simulink model "AVI_walking_SLIP"  (R2018a)
settings: Solver=ode45  StartTime=0.0  StopTime=100  MaxStep=1e-3  RelTol=1e-9  AbsTol=1e-6  EnableMultiTasking=on
values from neighbouring files (symbols this model uses):
  a_TD = 64.2076    [AVI_MatLabCode_REIERSEN.m]
  dx_0 = 1.06    [AVI_MatLabCode_REIERSEN.m]
  g = -9.81    [AVI_MatLabCode_REIERSEN.m]
  k = 10000    [AVI_MatLabCode_REIERSEN.m]
  l_0 = 1    [AVI_MatLabCode_REIERSEN.m]
  m = 80    [AVI_MatLabCode_REIERSEN.m]
  No_Steps = 25    [AVI_MatLabCode_REIERSEN.m]
  y_0 = 0.97    [AVI_MatLabCode_REIERSEN.m]
libraries: simulink x6, simulink_extras x1, dspswit3 x1
settings Model: Creator=Work  LastModifiedBy=gyrireiersen
settings SolverCC: AutoScaleAbsTol=off  ZeroCrossAlgorithm=Adaptive
settings DataIOCC: LimitDataPoints=on
settings OptimizationCC: LifeSpan=inf
settings DebuggingCC: AllowSymbolicDim=off  SFUnexpectedBacktrackingDiag=warning  SFNoUnconditionalDefaultTransitionDiag=warning  SFExecutionAtInitializationDiag=none
settings ModelReferenceCC: PropagateSignalLabelsOutOfModel=off
settings CodeAppCC: StateflowObjectComments=on
settings GRTTargetCC: TargetLangStandard=C89/C90 (ANSI)
settings ConfigComp: CovMetricSettings=dw  CovHtmlReporting=on  CovSaveCumulativeToWorkspaceVar=on  CovSaveSingleToWorkspaceVar=on  CovExternalEMLEnable=off

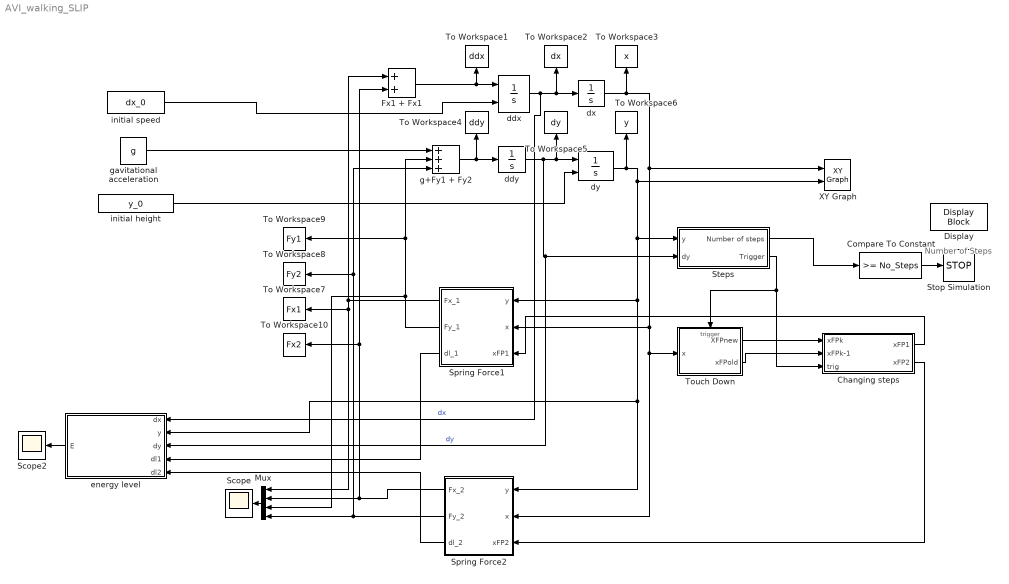
== system AVI_walking_SLIP ==
  note: Number of Steps
  Changing steps : Subsystem
  Compare To Constant : simulink/Logic and Bit Operations/Compare To Constant  relop=>=  const=No_Steps  OutDataTypeStr=boolean
  Display : DisplayBlock  WebBlockId=384  LabelPosition=Hide
  Fx1 + Fx1 : Sum
  Mux : Mux
  Scope : Scope
  Scope2 : Scope
  Spring Force1 : Subsystem
  Spring Force2 : Subsystem
  Steps : Subsystem
  Stop Simulation : Stop
  To Workspace1 : ToWorkspace  VariableName=ddx  SaveFormat=Timeseries  SampleTime=-1
  To Workspace10 : ToWorkspace  VariableName=Fx2  SaveFormat=Timeseries  SampleTime=-1
  To Workspace2 : ToWorkspace  VariableName=dx  SaveFormat=Timeseries  SampleTime=-1
  To Workspace3 : ToWorkspace  VariableName=x  SaveFormat=Timeseries  SampleTime=-1
  To Workspace4 : ToWorkspace  VariableName=ddy  SaveFormat=Timeseries  SampleTime=-1
  To Workspace5 : ToWorkspace  VariableName=dy  SaveFormat=Timeseries  SampleTime=-1
  To Workspace6 : ToWorkspace  VariableName=y  SaveFormat=Timeseries  SampleTime=-1
  To Workspace7 : ToWorkspace  VariableName=Fx1  SaveFormat=Timeseries  SampleTime=-1
  To Workspace8 : ToWorkspace  VariableName=Fy2  SaveFormat=Timeseries  SampleTime=-1
  To Workspace9 : ToWorkspace  VariableName=Fy1  SaveFormat=Timeseries  SampleTime=-1
  Touch Down : Subsystem
  XY Graph : simulink/Sinks/XY Graph  xmin=0  xmax=10  ymin=0  ymax=1.5  st=-1
  ddx : Integrator  InitialConditionSource=external
  ddy : Integrator
  dx : Integrator  LowerSaturationLimit=0
  dy : Integrator  InitialConditionSource=external  LimitOutput=on  LowerSaturationLimit=0
  energy level : Subsystem  TreatAsAtomicUnit=on
  g+Fy1 + Fy2 : Sum  Inputs=+++
  gavitational acceleration : Constant  Value=g
  initial height : Constant  Value=y_0
  initial speed : Constant  Value=dx_0
  wires:
  ddy/1 -> To Workspace5/1, dy/1, energy level/3(dy), Steps/2(dy)  "dy"
  ddx/1 -> To Workspace2/1, dx/1, energy level/1(dx)  "dx"
  gavitational acceleration/1 -> g+Fy1 + Fy2/1
  g+Fy1 + Fy2/1 -> To Workspace4/1, ddy/1
  initial speed/1 -> ddx/2
  initial height/1 -> dy/2
  dy/1 -> To Workspace6/1, Steps/1(y), Spring Force2/1(y), energy level/2(y), Spring Force1/1(y), XY Graph/2
  dx/1 -> Touch Down/1(x), Spring Force2/2(x), Spring Force1/2(x), XY Graph/1, To Workspace3/1
  Compare To Constant/1 -> Stop Simulation/1
  Changing steps/2(xFP2) -> Spring Force2/3(xFP2)
  Steps/1(Number of steps) -> Compare To Constant/1
  Steps/2("Trigger ") -> Touch Down/Trigger, Changing steps/3(trig)
  Touch Down/1(XFPnew) -> Changing steps/1(xFPk)
  Spring Force2/1(Fx_2) -> To Workspace10/1, Fx1 + Fx1/2, Mux/2
  Spring Force1/1(Fx_1) -> Fx1 + Fx1/1, To Workspace7/1, Mux/1
  Mux/1 -> Scope/1
  Changing steps/1(xFP1) -> Spring Force1/3(xFP1)
  Spring Force2/3(dl_2) -> energy level/5(dl2)
  energy level/1(E) -> Scope2/1
  Touch Down/2(xFPold) -> Changing steps/2(xFPk-1)
  Fx1 + Fx1/1 -> To Workspace1/1, ddx/1
  Spring Force1/3("dl_1 ") -> energy level/4(dl1)
  Spring Force2/2(Fy_2) -> To Workspace8/1, g+Fy1 + Fy2/3, Mux/4
  Spring Force1/2(Fy_1) -> Mux/3, g+Fy1 + Fy2/2, To Workspace9/1

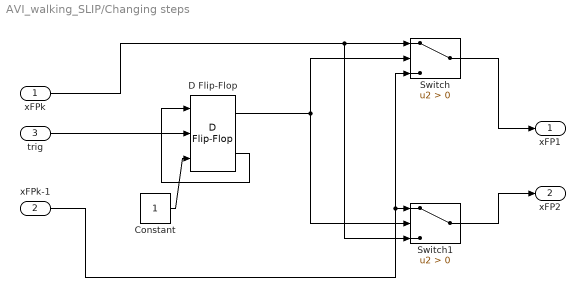
== system AVI_walking_SLIP/Changing steps ==
  xFPk : Inport
  xFPk-1 : Inport  Port=2
  trig : Inport  Port=3
  Constant : Constant
  D Flip-Flop : simulink_extras/Flip Flops/D Flip-Flop
      settings: SourceProductName=Simulink
  Switch : Switch  Criteria=u2 > Threshold
  Switch1 : Switch  Criteria=u2 > Threshold
  xFP1 : Outport
  xFP2 : Outport  Port=2
  wires:
  Constant/1 -> D Flip-Flop/3
  D Flip-Flop/2 -> D Flip-Flop/1
  trig/1 -> D Flip-Flop/2
  D Flip-Flop/1 -> Switch1/2, Switch/2
  xFPk/1 -> Switch1/3, Switch/1
  Switch/1 -> xFP1/1
  xFPk-1/1 -> Switch1/1, Switch/3
  Switch1/1 -> xFP2/1

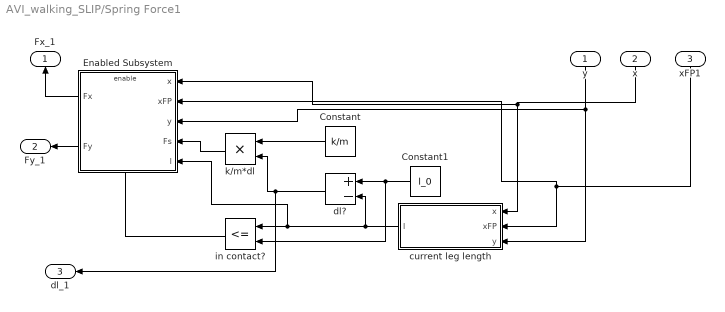
== system AVI_walking_SLIP/Spring Force1 ==
  y : Inport
  x : Inport  Port=2
  xFP1 : Inport  Port=3
  Constant : Constant  Value=k/m
  Constant1 : Constant  Value=l_0
  Enabled Subsystem : Subsystem  TreatAsAtomicUnit=on
  current leg length : Subsystem  TreatAsAtomicUnit=on
  dl? : Sum  Inputs=+-
  in contact? : RelationalOperator  Operator=<=  OutDataTypeStr=boolean  RndMeth=Nearest
  k/m*dl : Product
  Fx_1 : Outport
  Fy_1 : Outport  Port=2
  "dl_1 " : Outport  Port=3
  wires:
  xFP1/1 -> Enabled Subsystem/2(xFP), current leg length/2(xFP)
  x/1 -> Enabled Subsystem/1(x), current leg length/1(x)
  y/1 -> Enabled Subsystem/3(y), current leg length/3(y)
  k/m*dl/1 -> Enabled Subsystem/4(Fs)
  Enabled Subsystem/2(Fy) -> Fy_1/1
  current leg length/1(l) -> Enabled Subsystem/5(l), in contact?/1, dl?/2
  in contact?/1 -> Enabled Subsystem/Enable
  Enabled Subsystem/1(Fx) -> Fx_1/1
  dl?/1 -> "dl_1 "/1, k/m*dl/2
  Constant/1 -> k/m*dl/1
  Constant1/1 -> in contact?/2, dl?/1

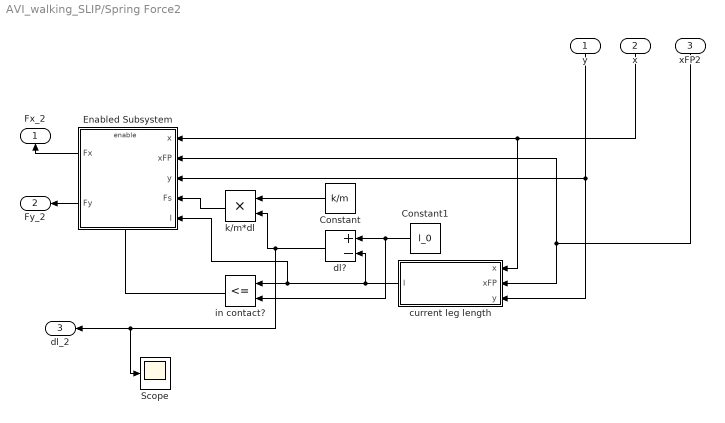
== system AVI_walking_SLIP/Spring Force2 ==
  y : Inport
  x : Inport  Port=2
  xFP2 : Inport  Port=3
  Constant : Constant  Value=k/m
  Constant1 : Constant  Value=l_0
  Enabled Subsystem : Subsystem  TreatAsAtomicUnit=on
  Scope : Scope
  current leg length : Subsystem  TreatAsAtomicUnit=on
  dl? : Sum  Inputs=+-
  in contact? : RelationalOperator  Operator=<=  OutDataTypeStr=boolean  RndMeth=Nearest
  k/m*dl : Product
  Fx_2 : Outport
  Fy_2 : Outport  Port=2
  dl_2 : Outport  Port=3
  wires:
  xFP2/1 -> Enabled Subsystem/2(xFP), current leg length/2(xFP)
  x/1 -> current leg length/1(x), Enabled Subsystem/1(x)
  y/1 -> Enabled Subsystem/3(y), current leg length/3(y)
  k/m*dl/1 -> Enabled Subsystem/4(Fs)
  Enabled Subsystem/2(Fy) -> Fy_2/1
  current leg length/1(l) -> Enabled Subsystem/5(l), in contact?/1, dl?/2
  in contact?/1 -> Enabled Subsystem/Enable
  dl?/1 -> Scope/1, dl_2/1, k/m*dl/2
  Enabled Subsystem/1(Fx) -> Fx_2/1
  Constant1/1 -> in contact?/2, dl?/1
  Constant/1 -> k/m*dl/1

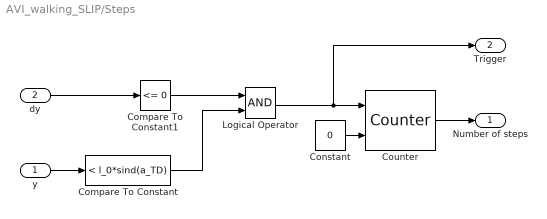
== system AVI_walking_SLIP/Steps ==
  y : Inport
  dy : Inport  Port=2
  Compare To Constant : simulink/Logic and Bit Operations/Compare To Constant  relop=<  const=l_0*sind(a_TD)  OutDataTypeStr=boolean
  Compare To Constant1 : simulink/Logic and Bit Operations/Compare To Constant  relop=<=  const=0  OutDataTypeStr=boolean
  Constant : Constant  Value=0
  Counter : dspswit3/Counter  Direction=Up  CountEvent=Rising edge  CounterSize=User defined  MaxCount=255  InitialCount=0  Output=Count  HitValue=32  ResetInput=on  SamplesPerFrame=1  Ts=1  CntDtype=single  HitDtype=Logical
  Logical Operator : Logic  AllPortsSameDT=off  OutDataTypeStr=boolean
  Number of steps : Outport
  "Trigger " : Outport  Port=2
  wires:
  Counter/1 -> Number of steps/1
  Compare To Constant/1 -> Logical Operator/2
  Logical Operator/1 -> "Trigger "/1, Counter/1
  Constant/1 -> Counter/2
  Compare To Constant1/1 -> Logical Operator/1
  dy/1 -> Compare To Constant1/1
  y/1 -> Compare To Constant/1

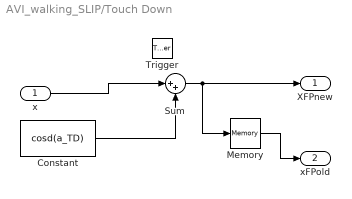
== system AVI_walking_SLIP/Touch Down ==
  x : Inport
  Trigger : TriggerPort  VariantControl=Variant  PortDimensions=1
  Constant : Constant  Value=cosd(a_TD)
  Memory : Memory  InheritSampleTime=on
  Sum : Sum  Inputs=|++
  XFPnew : Outport  InitialOutput=0
  xFPold : Outport  Port=2  InitialOutput=-1
  wires:
  x/1 -> Sum/1
  Memory/1 -> xFPold/1
  Sum/1 -> Memory/1, XFPnew/1
  Constant/1 -> Sum/2

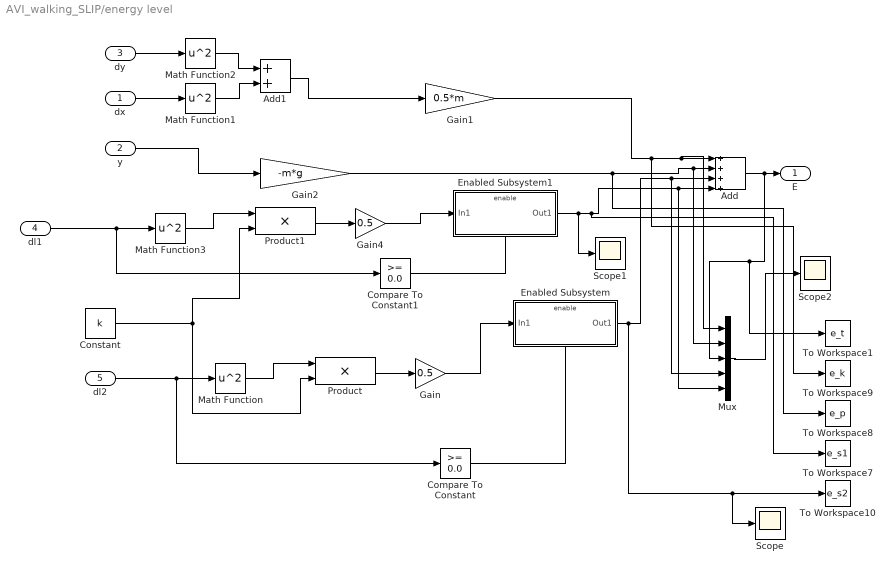
== system AVI_walking_SLIP/energy level ==
  dx : Inport
  y : Inport  Port=2
  dy : Inport  Port=3
  dl1 : Inport  Port=4
  dl2 : Inport  Port=5
  Add : Sum  Inputs=4
  Add1 : Sum  Inputs=2
  Compare To Constant : simulink/Logic and Bit Operations/Compare To Constant  relop=>=  const=0.0  OutDataTypeStr=boolean
  Compare To Constant1 : simulink/Logic and Bit Operations/Compare To Constant  relop=>=  const=0.0  OutDataTypeStr=boolean
  Constant : Constant  Value=k
  Enabled Subsystem : Subsystem  TreatAsAtomicUnit=on
  Enabled Subsystem1 : Subsystem  TreatAsAtomicUnit=on
  Gain : Gain  Gain=0.5
  Gain1 : Gain  Gain=0.5*m
  Gain2 : Gain  Gain=-m*g
  Gain4 : Gain  Gain=0.5
  Math Function{,1..3} (4 alike) : Math  Operator=square  SaturateOnIntegerOverflow=on
  Mux : Mux  Inputs=5
  Product : Product
  Product1 : Product
  Scope : Scope
  Scope1 : Scope
  Scope2 : Scope
  To Workspace1 : ToWorkspace  VariableName=e_t  SaveFormat=Timeseries  SampleTime=-1
  To Workspace10 : ToWorkspace  VariableName=e_s2  SaveFormat=Timeseries  SampleTime=-1
  To Workspace7 : ToWorkspace  VariableName=e_s1  SaveFormat=Timeseries  SampleTime=-1
  To Workspace8 : ToWorkspace  VariableName=e_p  SaveFormat=Timeseries  SampleTime=-1
  To Workspace9 : ToWorkspace  VariableName=e_k  SaveFormat=Timeseries  SampleTime=-1
  E : Outport
  wires:
  dx/1 -> Math Function1/1
  dl2/1 -> Compare To Constant/1, Math Function/1
  Math Function/1 -> Product/1
  Product/1 -> Gain/1
  y/1 -> Gain2/1
  Gain1/1 -> To Workspace9/1, Mux/1, Add/1
  Gain2/1 -> To Workspace8/1, Mux/2, Add/2
  Add/1 -> To Workspace1/1, Mux/3, E/1
  Gain/1 -> Enabled Subsystem/1(In1)
  Enabled Subsystem/1(Out1) -> Scope/1, To Workspace10/1, Mux/4, Add/3
  Compare To Constant/1 -> Enabled Subsystem/Enable
  Math Function2/1 -> Add1/1
  Math Function1/1 -> Add1/2
  Add1/1 -> Gain1/1
  dy/1 -> Math Function2/1
  Constant/1 -> Product/2, Product1/2
  Compare To Constant1/1 -> Enabled Subsystem1/Enable
  Math Function3/1 -> Product1/1
  Product1/1 -> Gain4/1
  Gain4/1 -> Enabled Subsystem1/1(In1)
  dl1/1 -> Compare To Constant1/1, Math Function3/1
  Enabled Subsystem1/1(Out1) -> Scope1/1, To Workspace7/1, Mux/5, Add/4
  Mux/1 -> Scope2/1

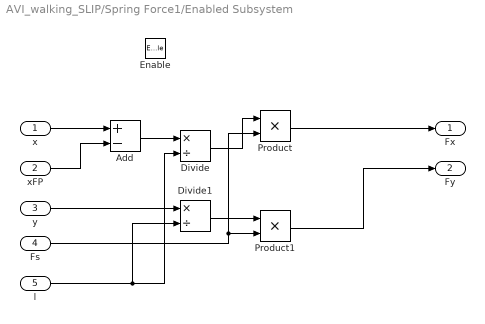
== system AVI_walking_SLIP/Spring Force1/Enabled Subsystem ==
  x : Inport
  xFP : Inport  Port=2
  y : Inport  Port=3
  Fs : Inport  Port=4
  l : Inport  Port=5
  Enable : EnablePort
  Add : Sum  Inputs=+-
  Divide : Product  Inputs=*/
  Divide1 : Product  Inputs=*/
  Product : Product
  Product1 : Product
  Fx : Outport
  Fy : Outport  Port=2
  wires:
  x/1 -> Add/1
  xFP/1 -> Add/2
  Add/1 -> Divide/1
  l/1 -> Divide1/2, Divide/2
  Divide/1 -> Product/1
  Fs/1 -> Product1/2, Product/2
  Product/1 -> Fx/1
  y/1 -> Divide1/1
  Divide1/1 -> Product1/1
  Product1/1 -> Fy/1

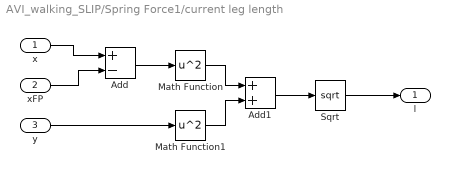
== system AVI_walking_SLIP/Spring Force1/current leg length ==
  x : Inport
  xFP : Inport  Port=2
  y : Inport  Port=3
  Add : Sum  Inputs=+-
  Add1 : Sum
  Math Function : Math  Operator=square  SaturateOnIntegerOverflow=on
  Math Function1 : Math  Operator=square  SaturateOnIntegerOverflow=on
  Sqrt : Sqrt  SaturateOnIntegerOverflow=on
  l : Outport
  wires:
  x/1 -> Add/1
  xFP/1 -> Add/2
  Add/1 -> Math Function/1
  y/1 -> Math Function1/1
  Math Function/1 -> Add1/1
  Math Function1/1 -> Add1/2
  Add1/1 -> Sqrt/1
  Sqrt/1 -> l/1

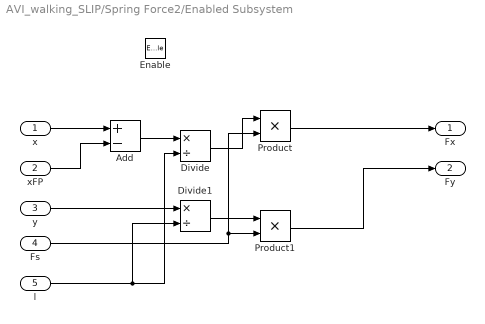
== system AVI_walking_SLIP/Spring Force2/Enabled Subsystem ==
  x : Inport
  xFP : Inport  Port=2
  y : Inport  Port=3
  Fs : Inport  Port=4
  l : Inport  Port=5
  Enable : EnablePort
  Add : Sum  Inputs=+-
  Divide : Product  Inputs=*/
  Divide1 : Product  Inputs=*/
  Product : Product
  Product1 : Product
  Fx : Outport
  Fy : Outport  Port=2
  wires:
  x/1 -> Add/1
  xFP/1 -> Add/2
  Add/1 -> Divide/1
  l/1 -> Divide1/2, Divide/2
  Divide/1 -> Product/1
  Fs/1 -> Product1/2, Product/2
  Product/1 -> Fx/1
  y/1 -> Divide1/1
  Divide1/1 -> Product1/1
  Product1/1 -> Fy/1

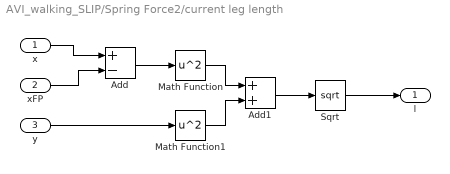
== system AVI_walking_SLIP/Spring Force2/current leg length ==
  x : Inport
  xFP : Inport  Port=2
  y : Inport  Port=3
  Add : Sum  Inputs=+-
  Add1 : Sum
  Math Function : Math  Operator=square  SaturateOnIntegerOverflow=on
  Math Function1 : Math  Operator=square  SaturateOnIntegerOverflow=on
  Sqrt : Sqrt  SaturateOnIntegerOverflow=on
  l : Outport
  wires:
  x/1 -> Add/1
  xFP/1 -> Add/2
  Add/1 -> Math Function/1
  y/1 -> Math Function1/1
  Math Function/1 -> Add1/1
  Math Function1/1 -> Add1/2
  Add1/1 -> Sqrt/1
  Sqrt/1 -> l/1

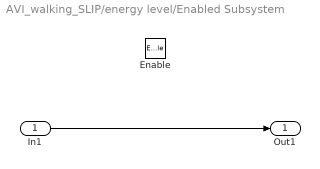
== system AVI_walking_SLIP/energy level/Enabled Subsystem ==
  In1 : Inport
  Enable : EnablePort
  Out1 : Outport
  wires:
  In1/1 -> Out1/1

== system AVI_walking_SLIP/energy level/Enabled Subsystem1 ==
  In1 : Inport
  Enable : EnablePort
  Out1 : Outport
  wires:
  In1/1 -> Out1/1
